simulink model "DataModelA"  (Simulink 10.0)
settings: Solver=FixedStepAuto  StartTime=0.0  StopTime=15  FixedStep=0.01  RelTol=1e-3
undefined symbols (not defined in the file): omega
libraries: fuzblock x4
settings Model: Creator=axs2437  LastModifiedBy=axs2437
settings DataIOCC: SaveFormat=Dataset
settings OptimizationCC: LifeSpan=auto
settings DebuggingCC: UnderspecifiedInitializationDetection=Simplified  MergeDetectMultiDrivingBlocksExec=error  SFUnexpectedBacktrackingDiag=error  SFNoUnconditionalDefaultTransitionDiag=error  SFExecutionAtInitializationDiag=warning  ArithmeticOperatorsInVariantConditions=error
settings HardwareCC: ProdBitPerPointer=64  ProdBitPerSizeT=64  ProdBitPerPtrDiffT=64  ProdLargestAtomicFloat=Float  ProdIntDivRoundTo=Zero  ProdEndianess=LittleEndian  ProdWordSize=64  ProdHWDeviceType=Intel->x86-64 (Windows64)
settings ModelReferenceCC: PropagateSignalLabelsOutOfModel=on
settings SFSimCC: SimUseLocalCustomCode=on  CustomCodeUndefinedFunction=FilterOut
settings RTWCC: RTWUseLocalCustomCode=on
settings CodeAppCC: StateflowObjectComments=off
settings GRTTargetCC: TargetLangStandard=C99 (ISO)  CombineOutputUpdateFcns=on  GRTInterface=off
settings ConfigComp: CovMetricSettings=dwe  CovHtmlReporting=off  CovSaveCumulativeToWorkspaceVar=off  CovSaveSingleToWorkspaceVar=off

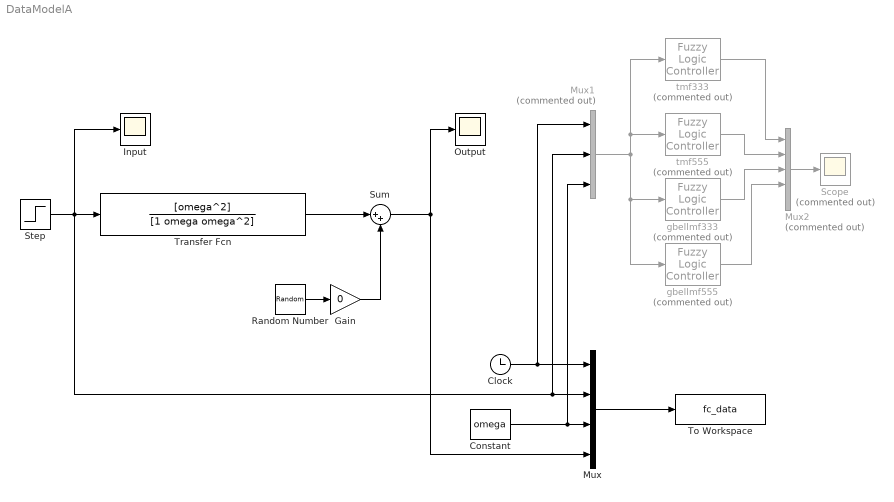
== system DataModelA ==
  Clock : Clock
  Constant : Constant  Value=omega
  Gain : Gain  Gain=0
  Input : Scope
  Mux : Mux
  Mux1 : Mux  Commented=on  Inputs=3
  Mux2 : Mux  Commented=on  Inputs=5
  Output : Scope
  Random Number : RandomNumber  Variance=0.001  SampleTime=0.01
  Scope : Scope  Commented=on
  Step : Step  SampleTime=0.01
  Sum : Sum  Inputs=|++
  To Workspace : ToWorkspace  VariableName=fc_data  SampleTime=-1
  Transfer Fcn : TransferFcn  Numerator=[omega^2]  Denominator=[1 omega omega^2]
  gbellmf333 : fuzblock/Fuzzy Logic  Controller  Commented=on  FIS=gbellmf333  OutputSampleNumber=101  DataType=double  FuzzifiedInputs=off  RuleFiringStrengths=off  RuleOutputs=off  AggregatedOutputs=off  SimulateUsing=Interpreted execution  OutOfRangeInputValueMessage=warning  NoRuleFiredMessage=warning  EmptyOutputFuzzySetMessage=warning
  gbellmf555 : fuzblock/Fuzzy Logic  Controller  Commented=on  FIS=gbellmf555  OutputSampleNumber=101  DataType=double  FuzzifiedInputs=off  RuleFiringStrengths=off  RuleOutputs=off  AggregatedOutputs=off  SimulateUsing=Interpreted execution  OutOfRangeInputValueMessage=warning  NoRuleFiredMessage=warning  EmptyOutputFuzzySetMessage=warning
  tmf333 : fuzblock/Fuzzy Logic  Controller  Commented=on  FIS=tmf333  OutputSampleNumber=101  DataType=double  FuzzifiedInputs=off  RuleFiringStrengths=off  RuleOutputs=off  AggregatedOutputs=off  SimulateUsing=Interpreted execution  OutOfRangeInputValueMessage=warning  NoRuleFiredMessage=warning  EmptyOutputFuzzySetMessage=warning
  tmf555 : fuzblock/Fuzzy Logic  Controller  Commented=on  FIS=tmf555  OutputSampleNumber=101  DataType=double  FuzzifiedInputs=off  RuleFiringStrengths=off  RuleOutputs=off  AggregatedOutputs=off  SimulateUsing=Interpreted execution  OutOfRangeInputValueMessage=warning  NoRuleFiredMessage=warning  EmptyOutputFuzzySetMessage=warning
  wires:
  gbellmf555/1 -> Mux2/4
  Clock/1 -> Mux1/1, Mux/1
  Constant/1 -> Mux1/3, Mux/3
  tmf555/1 -> Mux2/2
  tmf333/1 -> Mux2/1
  Random Number/1 -> Gain/1
  gbellmf333/1 -> Mux2/3
  Mux1/1 -> gbellmf555/1, gbellmf333/1, tmf333/1, tmf555/1
  Transfer Fcn/1 -> Sum/1
  Sum/1 -> Mux/4, Output/1
  Mux2/1 -> Scope/1
  Mux/1 -> To Workspace/1
  Gain/1 -> Sum/2
  Step/1 -> Input/1, Mux1/2, Mux/2, Transfer Fcn/1
